simulink model "gm_sampleModel1990_1_sub"  (R2023a)
settings: Solver=VariableStepAuto  StartTime=0.0  StopTime=10.0  RelTol=1e-3
libraries: simulink x1
settings Model: Creator=user1  LastModifiedBy=user1
settings OptimizationCC: BlockReduction=off  ConditionallyExecuteInputs=off
settings DebuggingCC: InheritedTsInSrcMsg=none

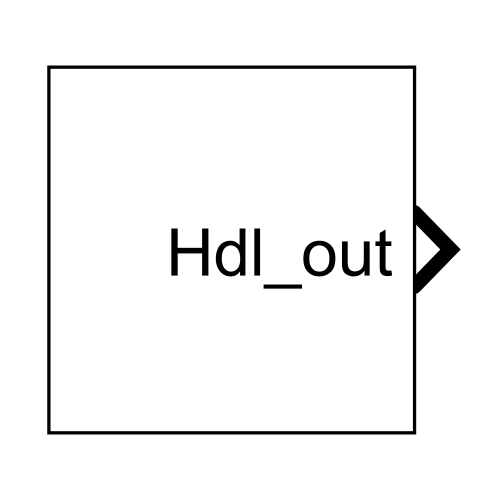
[thumbnail: Simulink's stored preview of the top-level diagram]
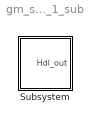
== system gm_sampleModel1990_1_sub ==
  Subsystem : Subsystem

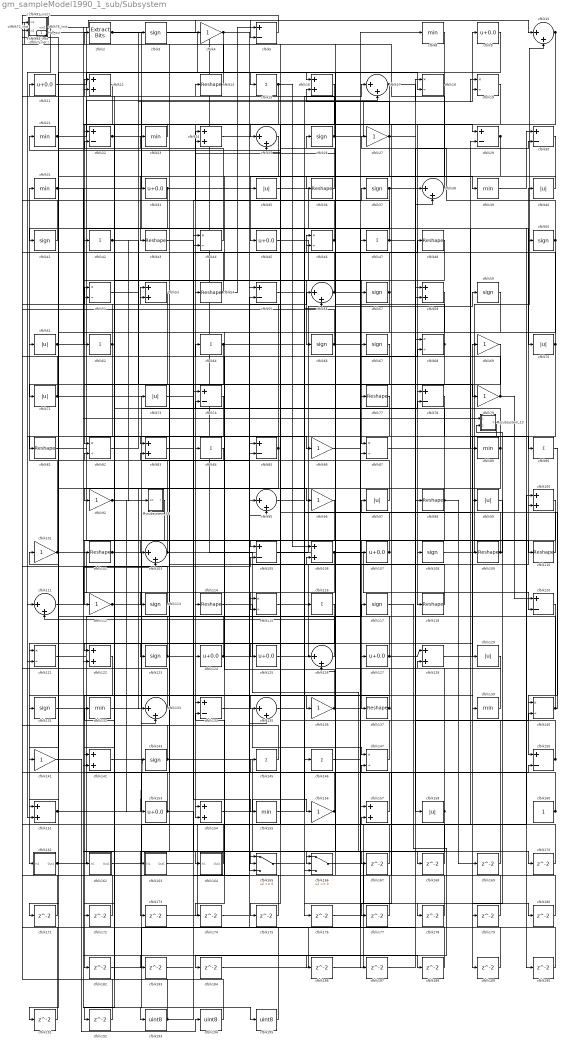
== system gm_sampleModel1990_1_sub/Subsystem ==
  Mysubsystem_13 : Subsystem
  Mysubsystem_34 : Subsystem
  cfblk{10,17,25,38,56,95,103,111,126,133,135} (11 alike) : Sum  Inputs=|++  OutDataTypeStr=uint8
  cfblk{12,16,24,53,58,83,100,106,122,128,142,151,154,157} (14 alike) : Sum  OutDataTypeStr=uint8
  cfblk{4,27,69,79,86,92,96,101,112,136,141,156} (12 alike) : Gain  OutDataTypeStr=uint8
  cfblk{14,36,43,48,54,77,81,98,102,109..110,114,118,137} (14 alike) : Reshape
  cfblk{5,22,29..30,55,74,78,85,105,120,134,150} (12 alike) : Sum  Inputs=+-  OutDataTypeStr=uint8
  cfblk{9,11,33,45,107,124..125,127,153} (9 alike) : Bias  Bias=0.0  SaturateOnIntegerOverflow=off
  cfblk{3,26,37,41,50,57,59,66..67,108,113,117,123,131,143} (15 alike) : Signum
  cfblk{18..19,44,46,52,68,82,87,115,121,140,147} (12 alike) : Product  Inputs=*/  OutDataTypeStr=uint8  RndMeth=Zero  SaturateOnIntegerOverflow=on
  cfblk{15,42,47,62,64,84,90,116,145..146} (10 alike) : Sum  Inputs=+  OutDataTypeStr=uint8
  cfblk119_inst : Subsystem
  cfblk{35,40,61,70..71,73,97,99,129,158} (10 alike) : Abs  OutDataTypeStr=uint8  SaturateOnIntegerOverflow=off
  cfblk130_inst : Subsystem
  cfblk{8,21,23,31,39,89,132,139,155} (9 alike) : MinMax  OutDataTypeStr=uint8
  cfblk138_inst : Subsystem
  cfblk13_inst : Subsystem
  cfblk144_inst : Subsystem
  cfblk148_inst : Subsystem
  cfblk149_inst : Subsystem
  cfblk152_inst : Subsystem
  cfblk160 : Constant  OutDataTypeStr=uint8  SampleTime=-1
  cfblk161 : Subsystem
  cfblk162 : Subsystem
  cfblk163 : Subsystem
  cfblk164 : Subsystem
  cfblk165 : Switch  OutDataTypeStr=uint8  SaturateOnIntegerOverflow=off  InputSameDT=off
  cfblk166 : Switch  OutDataTypeStr=uint8  SaturateOnIntegerOverflow=off  InputSameDT=off
  cfblk{167..180,182..184,186..192} (24 alike) : Delay  SampleTime=1
  cfblk193 : DataTypeConversion  OutDataTypeStr=uint8  SaturateOnIntegerOverflow=off  RndMeth=Floor
  cfblk194 : DataTypeConversion  OutDataTypeStr=uint8  SaturateOnIntegerOverflow=off  RndMeth=Floor
  cfblk195 : DataTypeConversion  OutDataTypeStr=uint8  SaturateOnIntegerOverflow=off  RndMeth=Floor
  cfblk2 : simulink/Logic and Bit Operations/Extract Bits  bitsToExtract=Upper half  numBits=8  bitIdxRange=[0 7]  outScalingMode=Preserve fixed-point scaling
      settings: LibrarySourceBlock=|
      | hdlsllib/Logic and Bit
      | Operations/Extract Bits
  cfblk28_inst : Subsystem
  cfblk32_inst : Subsystem
  cfblk34_inst : Subsystem
  cfblk49_inst : Subsystem
  cfblk51_inst : Subsystem
  cfblk60_inst : Subsystem
  cfblk63_inst : Subsystem
  cfblk65_inst : Subsystem
  cfblk6_inst : Subsystem
  cfblk72_inst : Subsystem
  cfblk76_inst : Subsystem
  cfblk7_inst : Subsystem
  cfblk91_inst : Subsystem
  cfblk94_inst : Subsystem
  Hdl_out : Outport  OutDataTypeStr=uint8  SampleTime=1
  wires:
  Mysubsystem_13/1(Out1) -> cfblk189/1
  Mysubsystem_34/1(Y) -> cfblk112/1
  cfblk10/1 -> cfblk154/2, cfblk118/1
  cfblk100/1 -> cfblk137/1
  cfblk101/1 -> cfblk154/1, cfblk31/1
  cfblk102/1 -> cfblk195/1, cfblk166/2
  cfblk103/1 -> cfblk72_inst/1(in1), cfblk106/2
  cfblk105/1 -> cfblk59/1
  cfblk106/1 -> cfblk124/1, cfblk120/2
  cfblk107/1 -> cfblk53/1, Hdl_out/1
  cfblk108/1 -> cfblk10/2
  cfblk109/1 -> cfblk152_inst/1(in1), cfblk130_inst/2(in2), Mysubsystem_13/2(In2)
  cfblk11/1 -> cfblk15/1
  cfblk110/1 -> cfblk97/1
  cfblk111/1 -> cfblk105/2
  cfblk112/1 -> cfblk133/2, cfblk136/1
  cfblk113/1 -> cfblk152_inst/2(in2)
  cfblk114/1 -> cfblk168/1
  cfblk115/1 -> cfblk176/1
  cfblk116/1 -> cfblk161/1(In1)
  cfblk117/1 -> cfblk184/1
  cfblk118/1 -> cfblk76_inst/2(in2)
  cfblk119_inst/1(out1) -> cfblk105/1
  cfblk12/1 -> cfblk82/1
  cfblk120/1 -> cfblk150/1
  cfblk121/1 -> cfblk117/1
  cfblk122/1 -> cfblk182/1
  cfblk123/1 -> cfblk48/1, cfblk144_inst/1(in1)
  cfblk124/1 -> cfblk65_inst/2(in2), cfblk40/1
  cfblk125/1 -> cfblk38/1
  cfblk126/1 -> cfblk51_inst/1(in1)
  cfblk127/1 -> cfblk128/1, cfblk52/1
  cfblk128/1 -> cfblk69/1
  cfblk129/1 -> cfblk128/2
  cfblk13_inst/1(out1) -> cfblk135/2
  cfblk130_inst/1(out1) -> cfblk66/1
  cfblk131/1 -> cfblk85/2
  cfblk132/1 -> cfblk74/2
  cfblk133/1 -> cfblk28_inst/1(in1)
  cfblk134/1 -> cfblk147/1
  cfblk135/1 -> cfblk17/1
  cfblk136/1 -> cfblk68/2, cfblk64/1
  cfblk137/1 -> cfblk72_inst/2(in2), cfblk131/1
  cfblk138_inst/1(out1) -> cfblk95/1, cfblk87/1
  cfblk139/1 -> cfblk7_inst/2(in2)
  cfblk14/1 -> cfblk13_inst/1(in1)
  cfblk140/1 -> cfblk61/1, cfblk100/2
  cfblk141/1 -> cfblk194/1
  cfblk142/1 -> cfblk188/1
  cfblk143/1 -> cfblk12/1, cfblk170/1
  cfblk144_inst/1(out1) -> cfblk55/1
  cfblk145/1 -> cfblk149_inst/2(in2)
  cfblk146/1 -> cfblk47/1
  cfblk147/1 -> cfblk2/1
  cfblk148_inst/1(out1) -> cfblk57/1
  cfblk149_inst/1(out1) -> cfblk32_inst/1(in1)
  cfblk15/1 -> cfblk25/1, cfblk106/1
  cfblk150/1 -> cfblk52/2, cfblk21/1
  cfblk151/1 -> cfblk143/1, cfblk116/1
  cfblk152_inst/1(out1) -> cfblk111/1
  cfblk153/1 -> cfblk165/2, cfblk101/1
  cfblk154/1 -> cfblk156/1
  cfblk155/1 -> cfblk99/1
  cfblk156/1 -> cfblk34_inst/2(in2), cfblk145/1
  cfblk157/1 -> cfblk148_inst/1(in1)
  cfblk158/1 -> cfblk111/2, cfblk173/1
  cfblk16/1 -> cfblk175/1
  cfblk160/1 -> cfblk53/2, cfblk148_inst/2(in2)
  cfblk161/1(Out1) -> cfblk67/1, cfblk150/2
  cfblk162/1(Out1) -> cfblk157/2
  cfblk163/1(Out1) -> cfblk44/1
  cfblk164/1(Out1) -> cfblk13_inst/2(in2)
  cfblk165/1 -> cfblk180/1
  cfblk166/1 -> cfblk178/1
  cfblk167/1 -> cfblk46/1
  cfblk168/1 -> cfblk25/2
  cfblk169/1 -> cfblk83/2
  cfblk17/1 -> cfblk158/1, cfblk172/1
  cfblk170/1 -> cfblk91_inst/1(in1)
  cfblk171/1 -> cfblk144_inst/2(in2)
  cfblk172/1 -> cfblk28_inst/2(in2)
  cfblk173/1 -> cfblk68/1
  cfblk174/1 -> cfblk56/1
  cfblk175/1 -> cfblk7_inst/1(in1)
  cfblk176/1 -> cfblk29/2
  cfblk177/1 -> cfblk134/2
  cfblk178/1 -> cfblk126/2
  cfblk179/1 -> cfblk147/2
  cfblk18/1 -> cfblk43/1, cfblk165/3, cfblk16/1
  cfblk180/1 -> cfblk60_inst/1(in1)
  cfblk182/1 -> cfblk87/2
  cfblk183/1 -> cfblk44/2
  cfblk184/1 -> cfblk38/2
  cfblk186/1 -> cfblk100/1
  cfblk187/1 -> cfblk140/2
  cfblk188/1 -> cfblk63_inst/1(in1)
  cfblk189/1 -> cfblk74/1
  cfblk19/1 -> cfblk167/1
  cfblk190/1 -> cfblk85/1
  cfblk191/1 -> cfblk138_inst/2(in2)
  cfblk192/1 -> cfblk49_inst/1(in1)
  cfblk193/1 -> cfblk65_inst/1(in1), cfblk165/1, cfblk130_inst/1(in1), cfblk132/1
  cfblk194/1 -> cfblk94_inst/1(in1)
  cfblk195/1 -> cfblk94_inst/2(in2)
  cfblk2/1 -> cfblk98/1, cfblk70/1
  cfblk21/1 -> cfblk56/2, cfblk17/2
  cfblk22/1 -> cfblk190/1, cfblk62/1
  cfblk23/1 -> cfblk22/1
  cfblk24/1 -> cfblk107/1
  cfblk25/1 -> cfblk81/1
  cfblk26/1 -> cfblk9/1, cfblk138_inst/1(in1)
  cfblk27/1 -> cfblk58/1, cfblk16/2, cfblk115/2
  cfblk28_inst/1(out1) -> cfblk166/3, cfblk125/1, cfblk10/1
  cfblk29/1 -> cfblk45/1, cfblk35/1
  cfblk3/1 -> cfblk18/2
  cfblk30/1 -> cfblk54/1
  cfblk31/1 -> cfblk19/2, cfblk187/1, cfblk146/1
  cfblk32_inst/1(out1) -> cfblk50/1, cfblk5/2
  cfblk33/1 -> cfblk95/2, cfblk192/1
  cfblk34_inst/1(out1) -> cfblk129/1
  cfblk35/1 -> cfblk89/1
  cfblk36/1 -> cfblk14/1
  cfblk37/1 -> cfblk58/2, cfblk41/1
  cfblk38/1 -> cfblk91_inst/2(in2)
  cfblk39/1 -> cfblk30/1
  cfblk4/1 -> cfblk151/1, cfblk39/1
  cfblk40/1 -> cfblk36/1
  cfblk41/1 -> cfblk49_inst/2(in2)
  cfblk42/1 -> cfblk79/1, Mysubsystem_34/1(In1)
  cfblk43/1 -> cfblk155/1
  cfblk44/1 -> cfblk11/1
  cfblk45/1 -> cfblk127/1
  cfblk46/1 -> cfblk51_inst/2(in2), cfblk26/1
  cfblk47/1 -> cfblk30/2, cfblk24/1
  cfblk48/1 -> cfblk102/1
  cfblk49_inst/1(out1) -> cfblk29/1, cfblk4/1
  cfblk5/1 -> cfblk119_inst/1(in1)
  cfblk50/1 -> cfblk27/1, cfblk177/1, cfblk171/1
  cfblk51_inst/1(out1) -> cfblk134/1, cfblk121/2
  cfblk52/1 -> cfblk3/1
  cfblk53/1 -> cfblk122/1
  cfblk54/1 -> cfblk63_inst/2(in2), cfblk5/1
  cfblk55/1 -> cfblk126/1
  cfblk56/1 -> cfblk32_inst/2(in2), cfblk8/1
  cfblk57/1 -> cfblk6_inst/2(in2), cfblk135/1
  cfblk58/1 -> cfblk164/1(In1)
  cfblk59/1 -> cfblk174/1
  cfblk6_inst/1(out1) -> cfblk113/1, cfblk183/1
  cfblk60_inst/1(out1) -> cfblk123/1
  cfblk61/1 -> cfblk33/1, cfblk109/1, cfblk86/1
  cfblk62/1 -> cfblk76_inst/1(in1), cfblk121/1
  cfblk63_inst/1(out1) -> cfblk103/1, cfblk96/1
  cfblk64/1 -> cfblk110/1, cfblk141/1
  cfblk65_inst/1(out1) -> cfblk42/1
  cfblk66/1 -> cfblk119_inst/2(in2), cfblk108/1
  cfblk67/1 -> cfblk122/2
  cfblk68/1 -> cfblk24/2, cfblk163/1(In1)
  cfblk69/1 -> cfblk78/1
  cfblk7_inst/1(out1) -> cfblk83/1, cfblk103/2
  cfblk70/1 -> cfblk6_inst/1(in1), cfblk151/2
  cfblk71/1 -> cfblk78/2, cfblk34_inst/1(in1)
  cfblk72_inst/1(out1) -> cfblk77/1, Mysubsystem_13/1(In1)
  cfblk73/1 -> cfblk139/1
  cfblk74/1 -> cfblk92/1
  cfblk76_inst/1(out1) -> cfblk186/1
  cfblk77/1 -> cfblk142/1
  cfblk78/1 -> cfblk84/1
  cfblk79/1 -> cfblk149_inst/1(in1), cfblk120/1
  cfblk8/1 -> cfblk166/1
  cfblk81/1 -> cfblk133/1
  cfblk82/1 -> cfblk19/1
  cfblk83/1 -> cfblk37/1
  cfblk84/1 -> cfblk82/2
  cfblk85/1 -> cfblk60_inst/2(in2), cfblk191/1
  cfblk86/1 -> cfblk157/1
  cfblk87/1 -> cfblk90/1
  cfblk89/1 -> cfblk46/2, cfblk115/1
  cfblk9/1 -> cfblk71/1
  cfblk90/1 -> cfblk140/1
  cfblk91_inst/1(out1) -> cfblk73/1
  cfblk92/1 -> cfblk55/2, cfblk22/2, cfblk153/1, cfblk162/1(In1)
  cfblk94_inst/1(out1) -> cfblk193/1
  cfblk95/1 -> cfblk18/1
  cfblk96/1 -> cfblk142/2
  cfblk97/1 -> cfblk23/1
  cfblk98/1 -> cfblk12/2, cfblk114/1, cfblk169/1
  cfblk99/1 -> cfblk179/1

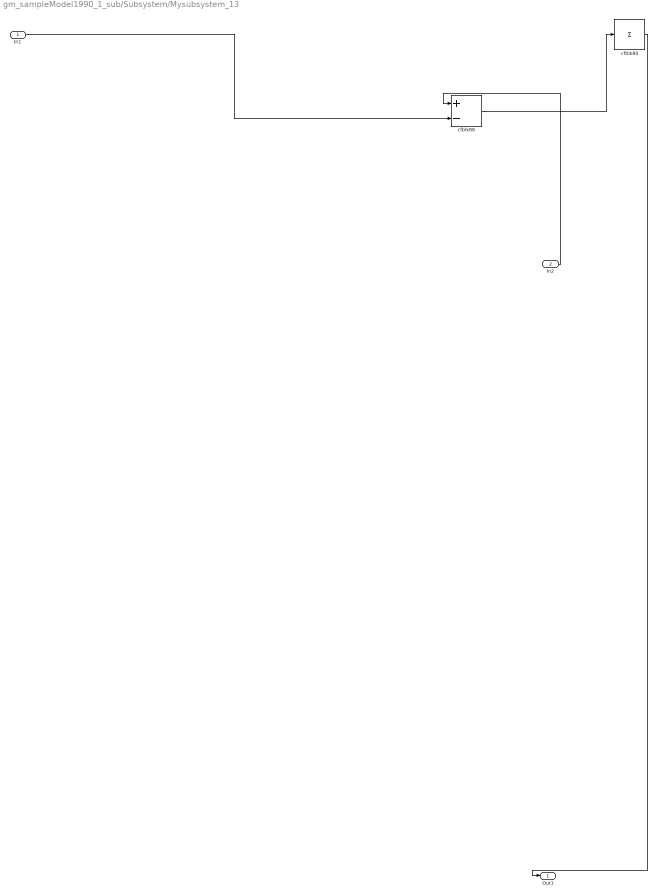
== system gm_sampleModel1990_1_sub/Subsystem/Mysubsystem_13 ==
  In1 : Inport  OutDataTypeStr=uint8  PortDimensions=1  SampleTime=1
  In2 : Inport  Port=2  OutDataTypeStr=uint8  PortDimensions=1  SampleTime=1
  cfblk80 : Sum  Inputs=+
  cfblk88 : Sum  Inputs=+-
  Out1 : Outport  SampleTime=1
  wires:
  In1/1 -> cfblk88/2
  In2/1 -> cfblk88/1
  cfblk80/1 -> Out1/1
  cfblk88/1 -> cfblk80/1

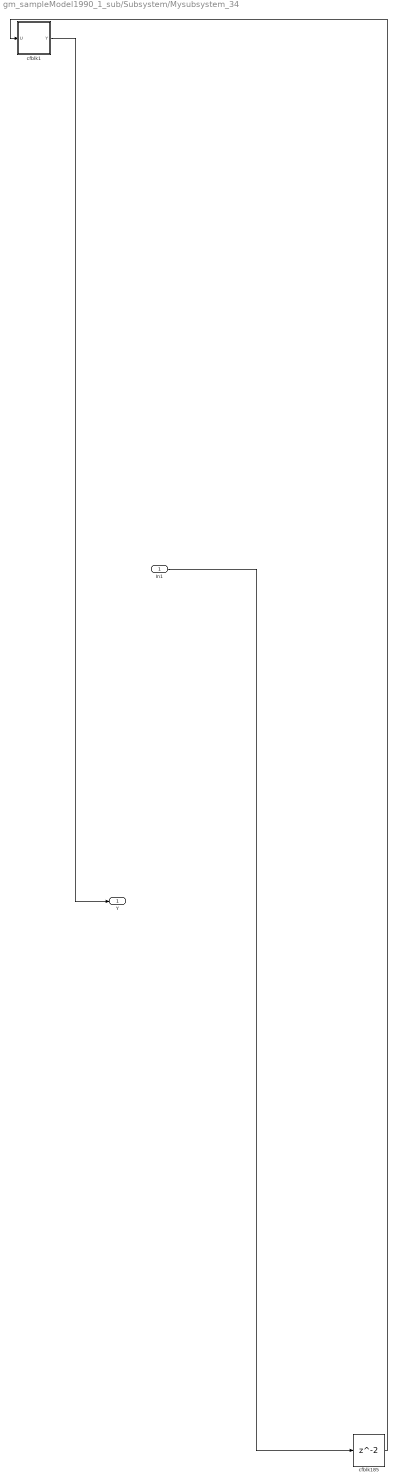
== system gm_sampleModel1990_1_sub/Subsystem/Mysubsystem_34 ==
  In1 : Inport  OutDataTypeStr=uint8  PortDimensions=1  SampleTime=1
  cfblk1 : Subsystem  mask(Detect Fall Negative){vinit=double(0), InputProcessing=Elements as channels (sample based), OutDataTypeStr=boolean}
      mask prompts: vinit "Simulink:masks:InitialCondition_MP"; InputProcessing "Simulink:masks:InputProcessing_MP"; OutDataTypeStr "Simulink:masks:OutputDataType_MP"
      mask help: Simulink:masks:DetectFallNegative_MD
      mask init:
      | InputProcessing = 'Elements as channels (sample based)';
      | OutDataTypeStr = 'boolean';
      | vinit = double(0);
      mask TypeOptions InputProcessing: Simulink:masks:ColumnsAsChannelsFrameBased | Simulink:masks:ElementsAsChannelsSampleBased
      mask TypeOptions OutDataTypeStr: Simulink:masks:uint8 | Simulink:masks:boolean
      mask Display: fprintf('U < 0\n&  NOT\nU/z < 0')
  cfblk185 : Delay  SampleTime=1
  Y : Outport  SampleTime=1
  wires:
  In1/1 -> cfblk185/1
  cfblk1/1(Y) -> Y/1
  cfblk185/1 -> cfblk1/1(U)

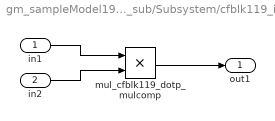
== system gm_sampleModel1990_1_sub/Subsystem/cfblk119_inst ==
  in1 : Inport  OutDataTypeStr=uint8  SampleTime=1
  in2 : Inport  Port=2  OutDataTypeStr=uint8  SampleTime=1
  mul_cfblk119_dotp_mulcomp : Product  Inputs=**  OutDataTypeStr=uint8  SampleTime=1
  out1 : Outport  OutDataTypeStr=uint8  SampleTime=1
  wires:
  in1/1 -> mul_cfblk119_dotp_mulcomp/1
  in2/1 -> mul_cfblk119_dotp_mulcomp/2
  mul_cfblk119_dotp_mulcomp/1 -> out1/1

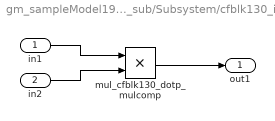
== system gm_sampleModel1990_1_sub/Subsystem/cfblk130_inst ==
  in1 : Inport  OutDataTypeStr=uint8  SampleTime=1
  in2 : Inport  Port=2  OutDataTypeStr=uint8  SampleTime=1
  mul_cfblk130_dotp_mulcomp : Product  Inputs=**  OutDataTypeStr=uint8  SampleTime=1
  out1 : Outport  OutDataTypeStr=uint8  SampleTime=1
  wires:
  in1/1 -> mul_cfblk130_dotp_mulcomp/1
  in2/1 -> mul_cfblk130_dotp_mulcomp/2
  mul_cfblk130_dotp_mulcomp/1 -> out1/1

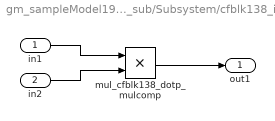
== system gm_sampleModel1990_1_sub/Subsystem/cfblk138_inst ==
  in1 : Inport  OutDataTypeStr=uint8  SampleTime=1
  in2 : Inport  Port=2  OutDataTypeStr=uint8  SampleTime=1
  mul_cfblk138_dotp_mulcomp : Product  Inputs=**  OutDataTypeStr=uint8  SampleTime=1
  out1 : Outport  OutDataTypeStr=uint8  SampleTime=1
  wires:
  in1/1 -> mul_cfblk138_dotp_mulcomp/1
  in2/1 -> mul_cfblk138_dotp_mulcomp/2
  mul_cfblk138_dotp_mulcomp/1 -> out1/1

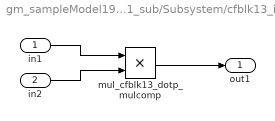
== system gm_sampleModel1990_1_sub/Subsystem/cfblk13_inst ==
  in1 : Inport  OutDataTypeStr=uint8  SampleTime=1
  in2 : Inport  Port=2  OutDataTypeStr=uint8  SampleTime=1
  mul_cfblk13_dotp_mulcomp : Product  Inputs=**  OutDataTypeStr=uint8  SampleTime=1
  out1 : Outport  OutDataTypeStr=uint8  SampleTime=1
  wires:
  in1/1 -> mul_cfblk13_dotp_mulcomp/1
  in2/1 -> mul_cfblk13_dotp_mulcomp/2
  mul_cfblk13_dotp_mulcomp/1 -> out1/1

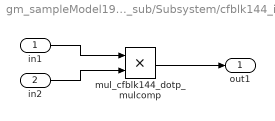
== system gm_sampleModel1990_1_sub/Subsystem/cfblk144_inst ==
  in1 : Inport  OutDataTypeStr=uint8  SampleTime=1
  in2 : Inport  Port=2  OutDataTypeStr=uint8  SampleTime=1
  mul_cfblk144_dotp_mulcomp : Product  Inputs=**  OutDataTypeStr=uint8  SampleTime=1
  out1 : Outport  OutDataTypeStr=uint8  SampleTime=1
  wires:
  in1/1 -> mul_cfblk144_dotp_mulcomp/1
  in2/1 -> mul_cfblk144_dotp_mulcomp/2
  mul_cfblk144_dotp_mulcomp/1 -> out1/1

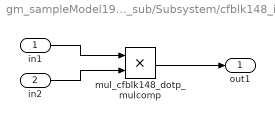
== system gm_sampleModel1990_1_sub/Subsystem/cfblk148_inst ==
  in1 : Inport  OutDataTypeStr=uint8  SampleTime=1
  in2 : Inport  Port=2  OutDataTypeStr=uint8  SampleTime=1
  mul_cfblk148_dotp_mulcomp : Product  Inputs=**  OutDataTypeStr=uint8  SampleTime=1
  out1 : Outport  OutDataTypeStr=uint8  SampleTime=1
  wires:
  in1/1 -> mul_cfblk148_dotp_mulcomp/1
  in2/1 -> mul_cfblk148_dotp_mulcomp/2
  mul_cfblk148_dotp_mulcomp/1 -> out1/1

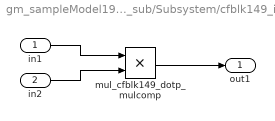
== system gm_sampleModel1990_1_sub/Subsystem/cfblk149_inst ==
  in1 : Inport  OutDataTypeStr=uint8  SampleTime=1
  in2 : Inport  Port=2  OutDataTypeStr=uint8  SampleTime=1
  mul_cfblk149_dotp_mulcomp : Product  Inputs=**  OutDataTypeStr=uint8  SampleTime=1
  out1 : Outport  OutDataTypeStr=uint8  SampleTime=1
  wires:
  in1/1 -> mul_cfblk149_dotp_mulcomp/1
  in2/1 -> mul_cfblk149_dotp_mulcomp/2
  mul_cfblk149_dotp_mulcomp/1 -> out1/1

== system gm_sampleModel1990_1_sub/Subsystem/cfblk152_inst ==
  in1 : Inport  OutDataTypeStr=uint8  SampleTime=1
  in2 : Inport  Port=2  OutDataTypeStr=uint8  SampleTime=1
  mul_cfblk152_dotp_mulcomp : Product  Inputs=**  OutDataTypeStr=uint8  SampleTime=1
  out1 : Outport  OutDataTypeStr=uint8  SampleTime=1
  wires:
  in1/1 -> mul_cfblk152_dotp_mulcomp/1
  in2/1 -> mul_cfblk152_dotp_mulcomp/2
  mul_cfblk152_dotp_mulcomp/1 -> out1/1

== system gm_sampleModel1990_1_sub/Subsystem/cfblk161 ==
  In1 : Inport  OutDataTypeStr=uint8  PortDimensions=1  SampleTime=1
  Out1 : Outport  SampleTime=1
  wires:
  In1/1 -> Out1/1

== system gm_sampleModel1990_1_sub/Subsystem/cfblk162 ==
  In1 : Inport  OutDataTypeStr=uint8  PortDimensions=1  SampleTime=1
  Out1 : Outport  SampleTime=1
  wires:
  In1/1 -> Out1/1

== system gm_sampleModel1990_1_sub/Subsystem/cfblk163 ==
  In1 : Inport  OutDataTypeStr=uint8  PortDimensions=1  SampleTime=1
  Out1 : Outport  SampleTime=1
  wires:
  In1/1 -> Out1/1

== system gm_sampleModel1990_1_sub/Subsystem/cfblk164 ==
  In1 : Inport  OutDataTypeStr=uint8  PortDimensions=1  SampleTime=1
  Out1 : Outport  SampleTime=1
  wires:
  In1/1 -> Out1/1

== system gm_sampleModel1990_1_sub/Subsystem/cfblk28_inst ==
  in1 : Inport  OutDataTypeStr=uint8  SampleTime=1
  in2 : Inport  Port=2  OutDataTypeStr=uint8  SampleTime=1
  mul_cfblk28_dotp_mulcomp : Product  Inputs=**  OutDataTypeStr=uint8  SampleTime=1
  out1 : Outport  OutDataTypeStr=uint8  SampleTime=1
  wires:
  in1/1 -> mul_cfblk28_dotp_mulcomp/1
  in2/1 -> mul_cfblk28_dotp_mulcomp/2
  mul_cfblk28_dotp_mulcomp/1 -> out1/1

== system gm_sampleModel1990_1_sub/Subsystem/cfblk32_inst ==
  in1 : Inport  OutDataTypeStr=uint8  SampleTime=1
  in2 : Inport  Port=2  OutDataTypeStr=uint8  SampleTime=1
  mul_cfblk32_dotp_mulcomp : Product  Inputs=**  OutDataTypeStr=uint8  SampleTime=1
  out1 : Outport  OutDataTypeStr=uint8  SampleTime=1
  wires:
  in1/1 -> mul_cfblk32_dotp_mulcomp/1
  in2/1 -> mul_cfblk32_dotp_mulcomp/2
  mul_cfblk32_dotp_mulcomp/1 -> out1/1

== system gm_sampleModel1990_1_sub/Subsystem/cfblk34_inst ==
  in1 : Inport  OutDataTypeStr=uint8  SampleTime=1
  in2 : Inport  Port=2  OutDataTypeStr=uint8  SampleTime=1
  mul_cfblk34_dotp_mulcomp : Product  Inputs=**  OutDataTypeStr=uint8  SampleTime=1
  out1 : Outport  OutDataTypeStr=uint8  SampleTime=1
  wires:
  in1/1 -> mul_cfblk34_dotp_mulcomp/1
  in2/1 -> mul_cfblk34_dotp_mulcomp/2
  mul_cfblk34_dotp_mulcomp/1 -> out1/1

== system gm_sampleModel1990_1_sub/Subsystem/cfblk49_inst ==
  in1 : Inport  OutDataTypeStr=uint8  SampleTime=1
  in2 : Inport  Port=2  OutDataTypeStr=uint8  SampleTime=1
  mul_cfblk49_dotp_mulcomp : Product  Inputs=**  OutDataTypeStr=uint8  SampleTime=1
  out1 : Outport  OutDataTypeStr=uint8  SampleTime=1
  wires:
  in1/1 -> mul_cfblk49_dotp_mulcomp/1
  in2/1 -> mul_cfblk49_dotp_mulcomp/2
  mul_cfblk49_dotp_mulcomp/1 -> out1/1

== system gm_sampleModel1990_1_sub/Subsystem/cfblk51_inst ==
  in1 : Inport  OutDataTypeStr=uint8  SampleTime=1
  in2 : Inport  Port=2  OutDataTypeStr=uint8  SampleTime=1
  mul_cfblk51_dotp_mulcomp : Product  Inputs=**  OutDataTypeStr=uint8  SampleTime=1
  out1 : Outport  OutDataTypeStr=uint8  SampleTime=1
  wires:
  in1/1 -> mul_cfblk51_dotp_mulcomp/1
  in2/1 -> mul_cfblk51_dotp_mulcomp/2
  mul_cfblk51_dotp_mulcomp/1 -> out1/1

== system gm_sampleModel1990_1_sub/Subsystem/cfblk60_inst ==
  in1 : Inport  OutDataTypeStr=uint8  SampleTime=1
  in2 : Inport  Port=2  OutDataTypeStr=uint8  SampleTime=1
  mul_cfblk60_dotp_mulcomp : Product  Inputs=**  OutDataTypeStr=uint8  SampleTime=1
  out1 : Outport  OutDataTypeStr=uint8  SampleTime=1
  wires:
  in1/1 -> mul_cfblk60_dotp_mulcomp/1
  in2/1 -> mul_cfblk60_dotp_mulcomp/2
  mul_cfblk60_dotp_mulcomp/1 -> out1/1

== system gm_sampleModel1990_1_sub/Subsystem/cfblk63_inst ==
  in1 : Inport  OutDataTypeStr=uint8  SampleTime=1
  in2 : Inport  Port=2  OutDataTypeStr=uint8  SampleTime=1
  mul_cfblk63_dotp_mulcomp : Product  Inputs=**  OutDataTypeStr=uint8  SampleTime=1
  out1 : Outport  OutDataTypeStr=uint8  SampleTime=1
  wires:
  in1/1 -> mul_cfblk63_dotp_mulcomp/1
  in2/1 -> mul_cfblk63_dotp_mulcomp/2
  mul_cfblk63_dotp_mulcomp/1 -> out1/1

== system gm_sampleModel1990_1_sub/Subsystem/cfblk65_inst ==
  in1 : Inport  OutDataTypeStr=uint8  SampleTime=1
  in2 : Inport  Port=2  OutDataTypeStr=uint8  SampleTime=1
  mul_cfblk65_dotp_mulcomp : Product  Inputs=**  OutDataTypeStr=uint8  SampleTime=1
  out1 : Outport  OutDataTypeStr=uint8  SampleTime=1
  wires:
  in1/1 -> mul_cfblk65_dotp_mulcomp/1
  in2/1 -> mul_cfblk65_dotp_mulcomp/2
  mul_cfblk65_dotp_mulcomp/1 -> out1/1

== system gm_sampleModel1990_1_sub/Subsystem/cfblk6_inst ==
  in1 : Inport  OutDataTypeStr=uint8  SampleTime=1
  in2 : Inport  Port=2  OutDataTypeStr=uint8  SampleTime=1
  mul_cfblk6_dotp_mulcomp : Product  Inputs=**  OutDataTypeStr=uint8  SampleTime=1
  out1 : Outport  OutDataTypeStr=uint8  SampleTime=1
  wires:
  in1/1 -> mul_cfblk6_dotp_mulcomp/1
  in2/1 -> mul_cfblk6_dotp_mulcomp/2
  mul_cfblk6_dotp_mulcomp/1 -> out1/1

== system gm_sampleModel1990_1_sub/Subsystem/cfblk72_inst ==
  in1 : Inport  OutDataTypeStr=uint8  SampleTime=1
  in2 : Inport  Port=2  OutDataTypeStr=uint8  SampleTime=1
  mul_cfblk72_dotp_mulcomp : Product  Inputs=**  OutDataTypeStr=uint8  SampleTime=1
  out1 : Outport  OutDataTypeStr=uint8  SampleTime=1
  wires:
  in1/1 -> mul_cfblk72_dotp_mulcomp/1
  in2/1 -> mul_cfblk72_dotp_mulcomp/2
  mul_cfblk72_dotp_mulcomp/1 -> out1/1

== system gm_sampleModel1990_1_sub/Subsystem/cfblk76_inst ==
  in1 : Inport  OutDataTypeStr=uint8  SampleTime=1
  in2 : Inport  Port=2  OutDataTypeStr=uint8  SampleTime=1
  mul_cfblk76_dotp_mulcomp : Product  Inputs=**  OutDataTypeStr=uint8  SampleTime=1
  out1 : Outport  OutDataTypeStr=uint8  SampleTime=1
  wires:
  in1/1 -> mul_cfblk76_dotp_mulcomp/1
  in2/1 -> mul_cfblk76_dotp_mulcomp/2
  mul_cfblk76_dotp_mulcomp/1 -> out1/1

== system gm_sampleModel1990_1_sub/Subsystem/cfblk7_inst ==
  in1 : Inport  OutDataTypeStr=uint8  SampleTime=1
  in2 : Inport  Port=2  OutDataTypeStr=uint8  SampleTime=1
  mul_cfblk7_dotp_mulcomp : Product  Inputs=**  OutDataTypeStr=uint8  SampleTime=1
  out1 : Outport  OutDataTypeStr=uint8  SampleTime=1
  wires:
  in1/1 -> mul_cfblk7_dotp_mulcomp/1
  in2/1 -> mul_cfblk7_dotp_mulcomp/2
  mul_cfblk7_dotp_mulcomp/1 -> out1/1

== system gm_sampleModel1990_1_sub/Subsystem/cfblk91_inst ==
  in1 : Inport  OutDataTypeStr=uint8  SampleTime=1
  in2 : Inport  Port=2  OutDataTypeStr=uint8  SampleTime=1
  mul_cfblk91_dotp_mulcomp : Product  Inputs=**  OutDataTypeStr=uint8  SampleTime=1
  out1 : Outport  OutDataTypeStr=uint8  SampleTime=1
  wires:
  in1/1 -> mul_cfblk91_dotp_mulcomp/1
  in2/1 -> mul_cfblk91_dotp_mulcomp/2
  mul_cfblk91_dotp_mulcomp/1 -> out1/1

== system gm_sampleModel1990_1_sub/Subsystem/cfblk94_inst ==
  in1 : Inport  OutDataTypeStr=uint8  SampleTime=1
  in2 : Inport  Port=2  OutDataTypeStr=uint8  SampleTime=1
  mul_cfblk94_dotp_mulcomp : Product  Inputs=**  OutDataTypeStr=uint8  SampleTime=1
  out1 : Outport  OutDataTypeStr=uint8  SampleTime=1
  wires:
  in1/1 -> mul_cfblk94_dotp_mulcomp/1
  in2/1 -> mul_cfblk94_dotp_mulcomp/2
  mul_cfblk94_dotp_mulcomp/1 -> out1/1

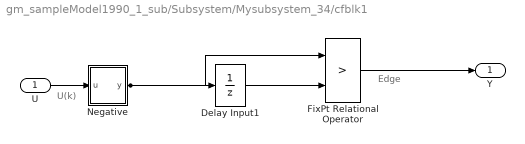
== system gm_sampleModel1990_1_sub/Subsystem/Mysubsystem_34/cfblk1 ==
  note: U(k)
  note: Edge
  U : Inport  OutDataTypeStr=uint8  SampleTime=1
  Delay Input1 : UnitDelay  Description=Store in Global RAM  DisableCoverage=on  InitialCondition=vinit  SampleTime=-1  HasFrameUpgradeWarning=on
  FixPt Relational Operator : RelationalOperator  Operator=>  OutDataTypeStr=boolean  ZeroCross=off  InputSameDT=off
  Negative : Subsystem  mask(Compare To Zero){relop=<, OutDataTypeStr=boolean, ZeroCross=off}
      mask prompts: relop "Simulink:masks:Operator_MP"; OutDataTypeStr "Simulink:masks:OutputDataType_MP"; ZeroCross "Simulink:masks:EnableZerocrossingDetection_MP"
      mask help: Simulink:masks:CompareToZero_MD
      mask init:
      | OutDataTypeStr = 'boolean';
      | ZeroCross = 'off';
      | blkName = 'sampleModel1990_1_sub/Subsystem/Mysubsystem_34/cfblk1/Negative';
      | relop = '<';
      | setValue = 'boolean';
      mask TypeOptions relop: == | ~= | < | <= | >= | >
      mask TypeOptions OutDataTypeStr: Simulink:masks:uint8 | Simulink:masks:boolean
      mask Callback ZeroCross: sl('zeroCrossEnable', gcbh);
      mask Display: disp([relop,' 0'])
  Y : Outport  SampleTime=1
  wires:
  U/1 -> Negative/1(u)
  Delay Input1/1 -> FixPt Relational Operator/2
  FixPt Relational Operator/1 -> Y/1
  Negative/1(y) -> FixPt Relational Operator/1, Delay Input1/1

== system gm_sampleModel1990_1_sub/Subsystem/Mysubsystem_34/cfblk1/Negative ==
  u : Inport  OutDataTypeStr=uint8  SampleTime=1
  Compare : RelationalOperator  Operator=<  OutDataTypeStr=boolean  ZeroCross=off
  Constant : Constant  DisableCoverage=on  Value=0  OutDataTypeStr=Inherit: Inherit via back propagation  SampleTime=-1  PreserveConstantTs=on
  y : Outport  SampleTime=1
  wires:
  u/1 -> Compare/1
  Compare/1 -> y/1
  Constant/1 -> Compare/2
